simulink model "Step_4_UR3_Data_Extraction"  (R2020a)
settings: Solver=ode3  StartTime=0.0  StopTime=10.0  FixedStep=0.001  RelTol=1e-3  EnableMultiTasking=on
settings Model: Creator=i7  LastModifiedBy=nnnmmm
settings DataIOCC: LimitDataPoints=on  SaveFormat=Array  ReturnWorkspaceOutputs=off
settings OptimizationCC: ExpressionDepthLimit=2147483647  LifeSpan=inf
settings DebuggingCC: UnderspecifiedInitializationDetection=Classic  MergeDetectMultiDrivingBlocksExec=none  SolverPrmCheckMsg=warning  FcnCallInpInsideContextMsg=warning  StateNameClashWarn=warning  SFUnexpectedBacktrackingDiag=warning  SFNoUnconditionalDefaultTransitionDiag=warning  SFExecutionAtInitializationDiag=none  ArithmeticOperatorsInVariantConditions=warning
settings HardwareCC: ProdBitPerPointer=32  ProdBitPerSizeT=32  ProdBitPerPtrDiffT=32  ProdLargestAtomicFloat=None  ProdIntDivRoundTo=Undefined  ProdEndianess=Unspecified  ProdWordSize=32  ProdHWDeviceType=32-bit Generic
settings ModelReferenceCC: PropagateSignalLabelsOutOfModel=off
settings SFSimCC: SimUseLocalCustomCode=off  CustomCodeUndefinedFunction=UseInterfaceOnly
settings RTWCC: RTWUseLocalCustomCode=off
settings CodeAppCC: StateflowObjectComments=on
settings GRTTargetCC: TargetLangStandard=C89/C90 (ANSI)  CombineOutputUpdateFcns=off  GRTInterface=on
settings ConfigComp: CovMetricSettings=dw  CovHtmlReporting=on  CovSaveCumulativeToWorkspaceVar=on  CovSaveSingleToWorkspaceVar=on  CovExternalEMLEnable=off

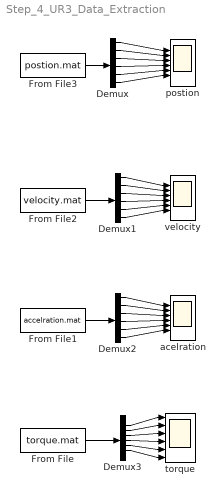
== system Step_4_UR3_Data_Extraction ==
  Demux{,1..3} (4 alike) : Demux  Outputs=6
  From File : FromFile  FileName=torque.mat  SampleTime=.1
  From File1 : FromFile  FileName=accelration.mat  SampleTime=.1
  From File2 : FromFile  FileName=velocity.mat  SampleTime=.1
  From File3 : FromFile  FileName=postion.mat  SampleTime=.1
  acelration : Scope  NumInputPorts=6
  postion : Scope  NumInputPorts=6
  torque : Scope  NumInputPorts=6
  velocity : Scope  NumInputPorts=6
  wires:
  Demux/1 -> postion/1
  Demux/2 -> postion/2
  Demux/3 -> postion/3
  Demux/4 -> postion/4
  Demux/5 -> postion/5
  Demux/6 -> postion/6
  Demux1/1 -> velocity/1
  Demux1/2 -> velocity/2
  Demux1/3 -> velocity/3
  Demux1/4 -> velocity/4
  Demux1/5 -> velocity/5
  Demux1/6 -> velocity/6
  Demux2/1 -> acelration/1
  Demux2/2 -> acelration/2
  Demux2/3 -> acelration/3
  Demux2/4 -> acelration/4
  Demux2/5 -> acelration/5
  Demux2/6 -> acelration/6
  Demux3/1 -> torque/1
  Demux3/2 -> torque/2
  Demux3/3 -> torque/3
  Demux3/4 -> torque/4
  Demux3/5 -> torque/5
  Demux3/6 -> torque/6
  From File/1 -> Demux3/1
  From File1/1 -> Demux2/1
  From File2/1 -> Demux1/1
  From File3/1 -> Demux/1
